simulink model "BLOCK_DIAGRAM_2"  (R2023b)
settings: Solver=VariableStepAuto  StartTime=0.0  StopTime=10.0  RelTol=1e-3
values from neighbouring files (symbols this model uses):
  G1_den = [1 0 0]    [BLOCK_DIAGRAM_2.m]    (also in untitled.m; untitled4.m)
  G1_num = [1]    [BLOCK_DIAGRAM_2.m]    (also in untitled.m; untitled4.m)
  G2_den = [1 1]    [BLOCK_DIAGRAM_2.m]    (also in untitled.m; untitled4.m)
  G2_num = [1]    [BLOCK_DIAGRAM_2.m]    (also in untitled.m; untitled4.m)
  G3_den = [1 0]    [BLOCK_DIAGRAM_2.m]    (also in untitled.m; untitled4.m)
  G3_num = [1]    [BLOCK_DIAGRAM_2.m]    (also in untitled.m; untitled4.m)
  G4_den = [2 0]    [BLOCK_DIAGRAM_2.m]    (also in untitled.m)
  G4_num = [1]    [BLOCK_DIAGRAM_2.m]    (also in untitled.m)
  H1_den = [1 0]    [BLOCK_DIAGRAM_2.m]    (also in untitled.m; untitled4.m)
  H1_num = [1]    [BLOCK_DIAGRAM_2.m]    (also in untitled.m; untitled4.m)
  H2_den = [1 -1]    [BLOCK_DIAGRAM_2.m]    (also in untitled.m; untitled4.m)
  H2_num = [1]    [BLOCK_DIAGRAM_2.m]    (also in untitled.m; untitled4.m)
  H3_den = [1 -2]    [BLOCK_DIAGRAM_2.m]    (also in untitled.m; untitled4.m)
  H3_num = [1]    [BLOCK_DIAGRAM_2.m]    (also in untitled.m; untitled4.m)
  Tf_den_final = [8 0 -32 -4 32 -8 -20 -8 -12 4 8 0 0 0 0 0 0 0]    [BLOCK_DIAGRAM_2.m]    (also in untitled.m = [1 0 -2 0 2 -1 -2 2 1 -1 0 0 0]; untitled4.m = [1 0 -2 0 2 -1 -2 2 1 -1 0 0 0])
  Tf_num_final = [4 -4 -12 4 8 0 0 0 0 0 0 0 0]    [BLOCK_DIAGRAM_2.m]    (also in untitled.m = [1 1 -5 -5 4 4 0 0 0 0]; untitled4.m = [1 1 -5 -5 4 4 0 0 0 0])
settings Model: Creator=Patrick James  LastModifiedBy=Patrick James

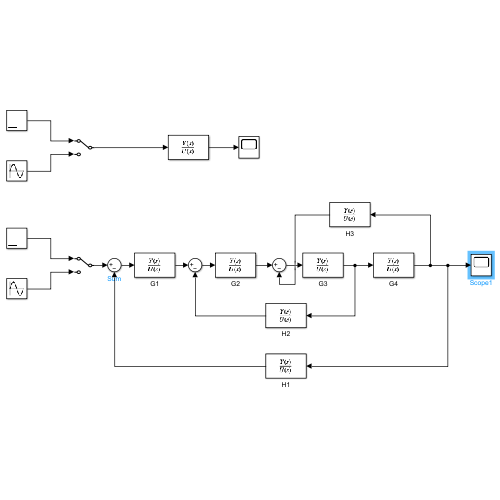
[thumbnail: Simulink's stored preview of the top-level diagram]
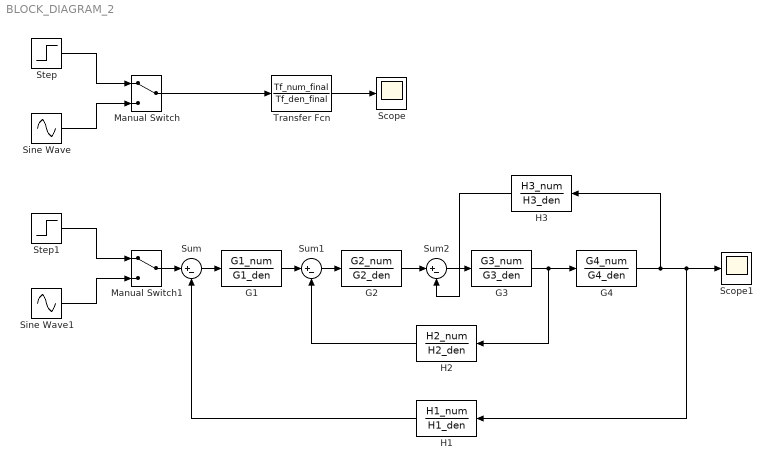
== system BLOCK_DIAGRAM_2 ==
  G1 : TransferFcn  Numerator=G1_num  Denominator=G1_den
  G2 : TransferFcn  Numerator=G2_num  Denominator=G2_den
  G3 : TransferFcn  Numerator=G3_num  Denominator=G3_den
  G4 : TransferFcn  Numerator=G4_num  Denominator=G4_den
  H1 : TransferFcn  Numerator=H1_num  Denominator=H1_den
  H2 : TransferFcn  Numerator=H2_num  Denominator=H2_den
  H3 : TransferFcn  Numerator=H3_num  Denominator=H3_den
  Manual Switch : ManualSwitch
  Manual Switch1 : ManualSwitch
  Scope : Scope
  Scope1 : Scope
  Sine Wave : Sin  SampleTime=0
  Sine Wave1 : Sin  SampleTime=0
  Step : Step  SampleTime=0
  Step1 : Step  SampleTime=0
  Sum : Sum  Inputs=|+-
  Sum1 : Sum  Inputs=|+-
  Sum2 : Sum  Inputs=|+-
  Transfer Fcn : TransferFcn  Numerator=Tf_num_final  Denominator=Tf_den_final
  wires:
  Transfer Fcn/1 -> Scope/1
  Step/1 -> Manual Switch/1
  Sine Wave/1 -> Manual Switch/2
  Manual Switch/1 -> Transfer Fcn/1
  Sine Wave1/1 -> Manual Switch1/2
  Step1/1 -> Manual Switch1/1
  Sum/1 -> G1/1
  Manual Switch1/1 -> Sum/1
  G1/1 -> Sum1/1
  Sum1/1 -> G2/1
  G2/1 -> Sum2/1
  Sum2/1 -> G3/1
  G3/1 -> H2/1, G4/1
  H3/1 -> Sum2/2
  G4/1 -> H1/1, Scope1/1, H3/1
  H2/1 -> Sum1/2
  H1/1 -> Sum/2
